simulink model "bramBurst_TransposeMatrix"  (R2021a)
settings: Solver=FixedStepDiscrete  StartTime=0.0  StopTime=44550*Ts  RelTol=1e-3
InitFcn:
  | matched_filter_fft_hdl_init;
model workspace (MAT data in the model file):
  mwTaskManagerKernelLatency = 0
  socvcb : containers.Map (value not decoded)
undefined symbols (not defined in the file or in its folder): columnWindowFun, DTsig_in, DTWindowFun, hdlbramBurst, N1, N2, radarDataCube, Ts
libraries: hdlsllib x35, simulink x11, dsphdlxfrm x1, dsphdlfiltering x1
(part 2 of 2)

== system bramBurst_TransposeMatrix/XDF/MatrixTranspose/addressControl/DDRbaseAddrCalc ==
  baseAddr : Inport
  ddrBank : Inport  Port=2
  Add : Sum  OutDataTypeStr=uint32
  Constant : Constant  Value=(N1 * N2 * hdlbramBurst.pAXIDataWidthBytes)  OutDataTypeStr=uint32  SampleTime=-1
  Switch1 : Switch  Criteria=u2 ~= 0
  Switch2 : Switch  Criteria=u2 ~= 0
  ddrWrAddr : Outport
  ddrRdAddr : Outport  Port=2
  wires:
  Constant/1 -> Add/1
  Add/1 -> Switch2/3, Switch1/1
  Switch1/1 -> ddrWrAddr/1
  ddrBank/1 -> Switch2/2, Switch1/2
  baseAddr/1 -> Switch2/1, Switch1/3, Add/2
  Switch2/1 -> ddrRdAddr/1

== system bramBurst_TransposeMatrix/XDF/MatrixTranspose/addressControl/ping_pong ==
  note: if 0 is selected then use first bank (starting at address 0) to read from
      | if 1 is selected then use the second bank (starting at offset) to read from
  ddrDone : Inport
  Logical Operator9 : Logic  Operator=XOR  IconShape=distinctive  AllPortsSameDT=off  OutDataTypeStr=boolean
  Unit Delay1 : UnitDelay  SampleTime=-1  HasFrameUpgradeWarning=on
  sr_latch : Subsystem
  ddrBank : Outport  VectorParamsAs1DForOutWhenUnconnected=off
  wires:
  Unit Delay1/1 -> Logical Operator9/1
  Logical Operator9/1 -> sr_latch/1(S)
  ddrDone/1 -> sr_latch/2(R), Logical Operator9/2
  sr_latch/1(Q) -> Unit Delay1/1, ddrBank/1  "DDR_BankSelect"

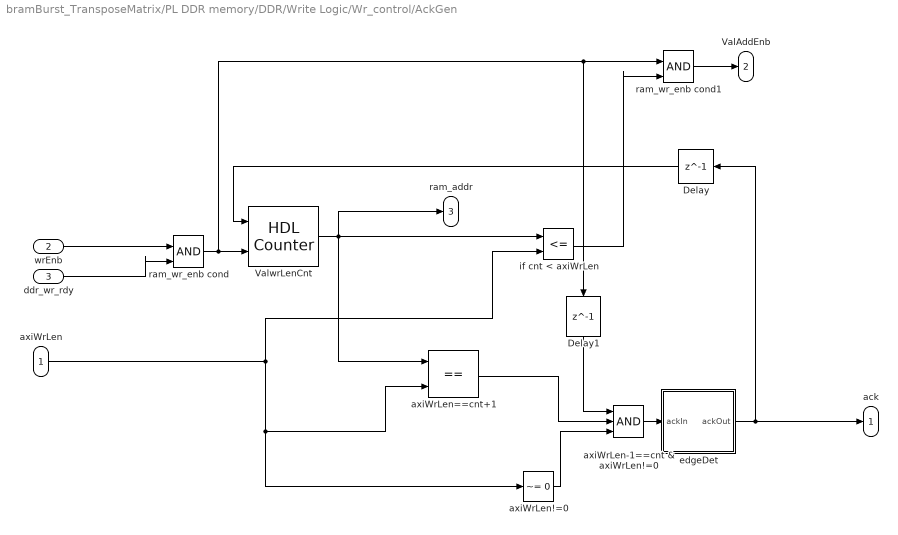
== system bramBurst_TransposeMatrix/PL DDR memory/DDR/Write Logic/Wr_control/AckGen ==
  axiWrLen : Inport
  wrEnb : Inport  Port=2
  ddr_wr_rdy : Inport  Port=3
  Delay : Delay  DelayLength=1
  Delay1 : Delay  DelayLength=1
  ValwrLenCnt : hdlsllib/Sources/HDL Counter  CountType=Free running  CountInit=0  CountStep=1  CountMax=25  CountFromType=Initial value  CountFrom=0  CountResetPort=on  CountLoadPort=off  CountEnbPort=on  CountDirPort=off  CountHitOutputPort=off  CountDataType=Unsigned  CountWordLen=32  CountFracLen=0  CountSampTime=1
  axiWrLen!=0 : simulink/Logic and Bit Operations/Compare To Constant  relop=~=  const=0  OutDataTypeStr=boolean
  "axiWrLen-1==cnt & axiWrLen!=0 " : Logic  Inputs=3  IconShape=distinctive  AllPortsSameDT=off  OutDataTypeStr=boolean
  axiWrLen==cnt+1 : RelationalOperator  Operator===  OutDataTypeStr=boolean  RndMeth=Nearest
  edgeDet : Subsystem
  if cnt < axiWrLen : RelationalOperator  Operator=<=  OutDataTypeStr=boolean  RndMeth=Nearest
  ram_wr_enb cond : Logic  IconShape=distinctive  AllPortsSameDT=off  OutDataTypeStr=boolean
  ram_wr_enb cond1 : Logic  IconShape=distinctive  AllPortsSameDT=off  OutDataTypeStr=boolean
  ack : Outport  VectorParamsAs1DForOutWhenUnconnected=off
  ValAddEnb : Outport  Port=2  VectorParamsAs1DForOutWhenUnconnected=off
  ram_addr : Outport  Port=3  VectorParamsAs1DForOutWhenUnconnected=off
  wires:
  Delay1/1 -> "axiWrLen-1==cnt & axiWrLen!=0 "/1
  Delay/1 -> ValwrLenCnt/1
  ram_wr_enb cond1/1 -> ValAddEnb/1
  ram_wr_enb cond/1 -> ValwrLenCnt/2, Delay1/1, ram_wr_enb cond1/1
  ddr_wr_rdy/1 -> ram_wr_enb cond/2
  ValwrLenCnt/1 -> ram_addr/1, if cnt < axiWrLen/1, axiWrLen==cnt+1/1
  axiWrLen/1 -> if cnt < axiWrLen/2, axiWrLen!=0/1, axiWrLen==cnt+1/2
  if cnt < axiWrLen/1 -> ram_wr_enb cond1/2
  wrEnb/1 -> ram_wr_enb cond/1
  axiWrLen!=0/1 -> "axiWrLen-1==cnt & axiWrLen!=0 "/3
  axiWrLen==cnt+1/1 -> "axiWrLen-1==cnt & axiWrLen!=0 "/2
  edgeDet/1(ackOut) -> Delay/1, ack/1
  "axiWrLen-1==cnt & axiWrLen!=0 "/1 -> edgeDet/1(ackIn)

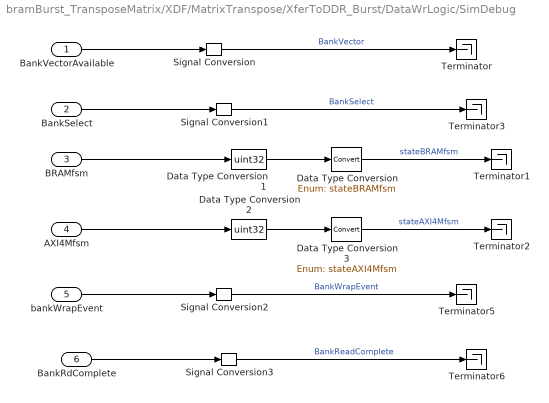
== system bramBurst_TransposeMatrix/XDF/MatrixTranspose/XferToDDR_Burst/DataWrLogic/SimDebug ==
  BankVectorAvailable : Inport
  BankSelect : Inport  Port=2
  BRAMfsm : Inport  Port=3
  AXI4Mfsm : Inport  Port=4
  bankWrapEvent : Inport  Port=5
  BankRdComplete : Inport  Port=6
  Data Type Conversion : DataTypeConversion  OutDataTypeStr=Enum: stateBRAMfsm
  Data Type Conversion1 : DataTypeConversion  OutDataTypeStr=uint32
  Data Type Conversion2 : DataTypeConversion  OutDataTypeStr=uint32
  Data Type Conversion3 : DataTypeConversion  OutDataTypeStr=Enum: stateAXI4Mfsm
  Signal Conversion{,1..3} (4 alike) : SignalConversion  OverrideOpt=off
  Terminator{,1..3,5..6} (6 alike) : Terminator
  wires:
  Signal Conversion/1 -> Terminator/1  "BankVector"
  Data Type Conversion2/1 -> Data Type Conversion3/1
  Data Type Conversion3/1 -> Terminator2/1  "stateAXI4Mfsm"
  Signal Conversion2/1 -> Terminator5/1  "BankWrapEvent"
  Data Type Conversion1/1 -> Data Type Conversion/1
  Signal Conversion3/1 -> Terminator6/1  "BankReadComplete"
  Signal Conversion1/1 -> Terminator3/1  "BankSelect"
  Data Type Conversion/1 -> Terminator1/1  "stateBRAMfsm"
  BRAMfsm/1 -> Data Type Conversion1/1
  AXI4Mfsm/1 -> Data Type Conversion2/1
  BankVectorAvailable/1 -> Signal Conversion/1
  bankWrapEvent/1 -> Signal Conversion2/1
  BankRdComplete/1 -> Signal Conversion3/1
  BankSelect/1 -> Signal Conversion1/1

== system bramBurst_TransposeMatrix/XDF/MatrixTranspose/XferToDDR_Burst/DataWrLogic/Subsystem ==
  wrctrlOut : Inport
  bankRdComplete : Inport  Port=2
  FIFO_backpressure_applied : Inport  Port=3
  <wr_complete> : Inport  Port=4
  In5 : Inport  Port=5
  Bit Concat : hdlsllib/Logic and Bit Operations/Bit Concat  numInputs=2
  Bus Selector1 : BusSelector  OutputSignals=wr_valid
  DebugBus : BusCreator  Inputs=5
  Demux : Demux  Outputs=2
  Detect Increase : simulink/Logic and Bit Operations/Detect Increase  vinit=0.0  OutDataTypeStr=boolean
  HDL Counter{,1..3} (4 alike) : hdlsllib/Sources/HDL Counter  CountType=Free running  CountInit=0  CountStep=1  CountMax=25  CountFromType=Initial value  CountFrom=0  CountResetPort=off  CountLoadPort=off  CountEnbPort=on  CountDirPort=off  CountHitOutputPort=off  CountDataType=Unsigned  CountWordLen=32  CountFracLen=0  CountSampTime=1
  Logical Operator1 : Logic  Operator=NOT  AllPortsSameDT=off  OutDataTypeStr=boolean
  debugRd : Outport
  wires:
  wrctrlOut/1 -> Bus Selector1/1
  FIFO_backpressure_applied/1 -> Logical Operator1/1
  HDL Counter2/1 -> DebugBus/1  "wr_complete_counter"
  <wr_complete>/1 -> HDL Counter2/1
  bankRdComplete/1 -> Detect Increase/1
  DebugBus/1 -> debugRd/1
  HDL Counter3/1 -> DebugBus/2  "bankCompleteCounter"
  Logical Operator1/1 -> HDL Counter/1
  HDL Counter/1 -> DebugBus/3  "FIFO_back_pressure_applied"
  Bus Selector1/1 -> HDL Counter1/1  "<wr_valid>"
  Detect Increase/1 -> HDL Counter3/1
  HDL Counter1/1 -> DebugBus/4  "CountWriteValids"
  In5/1 -> Demux/1
  Demux/1 -> Bit Concat/1
  Demux/2 -> Bit Concat/2
  Bit Concat/1 -> DebugBus/5  "FSM_read"

== system bramBurst_TransposeMatrix/XDF/MatrixTranspose/addressControl/ping_pong/sr_latch ==
  S : Inport
  R : Inport  Port=2
  Logical Operator1 : Logic  IconShape=distinctive  AllPortsSameDT=off  OutDataTypeStr=boolean
  Logical Operator2 : Logic  Operator=NOT  IconShape=distinctive  AllPortsSameDT=off  OutDataTypeStr=boolean
  Logical Operator9 : Logic  Operator=OR  IconShape=distinctive  AllPortsSameDT=off  OutDataTypeStr=boolean
  Unit Delay1 : UnitDelay  SampleTime=-1  HasFrameUpgradeWarning=on
  Q : Outport  VectorParamsAs1DForOutWhenUnconnected=off
  wires:
  Logical Operator9/1 -> Q/1, Unit Delay1/1
  Unit Delay1/1 -> Logical Operator1/2
  S/1 -> Logical Operator9/1
  R/1 -> Logical Operator2/1
  Logical Operator2/1 -> Logical Operator1/1
  Logical Operator1/1 -> Logical Operator9/2

== system bramBurst_TransposeMatrix/PL DDR memory/DDR/Write Logic/Wr_control/AckGen/edgeDet ==
  ackIn : Inport
  " ackIn==1" : simulink/Logic and Bit Operations/Compare To Constant  relop===  const=1  OutDataTypeStr=boolean
  ackIn Posedge Detect : Logic  IconShape=distinctive  AllPortsSameDT=off  OutDataTypeStr=boolean
  ackIn_d1 : Delay  DelayLength=1
  ackIn_d1==0 : simulink/Logic and Bit Operations/Compare To Constant  relop===  const=0  OutDataTypeStr=boolean
  ackOut : Outport  VectorParamsAs1DForOutWhenUnconnected=off
  wires:
  ackIn/1 -> ackIn_d1/1, " ackIn==1"/1
  ackIn_d1/1 -> ackIn_d1==0/1
  ackIn Posedge Detect/1 -> ackOut/1
  ackIn_d1==0/1 -> ackIn Posedge Detect/1
  " ackIn==1"/1 -> ackIn Posedge Detect/2

== matlab function bramBurst_TransposeMatrix/PL DDR memory/DDR/DDR Memory ==
  data: wr_din input INTERFACE_DT size=[INTERFACE_NUM_WORDS 1]; rd_dout output INTERFACE_DT size=[1 INTERFACE_NUM_WORDS]; wr_addr input; wr_en input; rd_addr input; INIT_DATA parameter; DDR_SIZE parameter; INIT_ADDR parameter; INTERFACE_WORD_LENGTH parameter; mem_data output; INTERFACE_NUM_WORDS parameter
function [rd_dout, mem_data] = ddr_memory(wr_din,wr_addr,wr_en,rd_addr,...
    INIT_DATA, DDR_SIZE, INIT_ADDR, INTERFACE_WORD_LENGTH, INTERFACE_NUM_WORDS)

DATA_NUM_BYTES = dataNumBytes(wr_din);

persistent mem
if isempty(mem)
    mem = zeros([1 DDR_SIZE],'uint8');
    if ~isempty(INIT_DATA)
        init_data_u8 = dataToBytes(INIT_DATA);
        idx = (1:numel(init_data_u8)) + INIT_ADDR;
        mem(idx) = init_data_u8;
    end
end

persistent rd_dout_reg
if isempty(rd_dout_reg)
    rd_dout_reg = zeros([1 INTERFACE_NUM_WORDS],'like',wr_din);
end

rd_dout = rd_dout_reg;

% READ update
rd_idx = (1:DATA_NUM_BYTES) + double(rd_addr);
if (rd_idx(end) > DDR_SIZE)
    error('Read from address 0x%X exceeds memory size.',uint32(rd_addr))
end
mem_rd_bytes = mem(rd_idx);
rd_dout_temp = zeros([1 INTERFACE_NUM_WORDS],'like',wr_din);
rd_dout_temp(:) = bytesToData(mem_rd_bytes, coder.const(INTERFACE_WORD_LENGTH));
% bytesToData
% if INTERFACE_WORD_LENGTH == 128
%     temp = typecast(mem_rd_bytes,'uint64');
%     temp1 = reshape(temp,2,[]);
%     rd_dout_temp(:)  = sim2fi(temp1, 0,128,0);
% else
%     rd_dout_temp(:)  = typecast(mem_rd_bytes,sprintf('uint%d',INTERFACE_WORD_LENGTH));
% end

rd_dout_reg = rd_dout_temp;

% WRITE update
if wr_en
    wr_idx = (1:DATA_NUM_BYTES) + double(wr_addr);
    if (wr_idx(end) > DDR_SIZE)
        error('Write from address 0x%X exceeds memory size.',uint32(wr_addr))
    end
    mem(wr_idx) = dataToBytes(wr_din);
end

mem_data = mem;

end

function dout = dataToBytes(din)
    temp1 = reshape(din,[],1); % force column vector
    if isfi(din)
        temp2 = reshape(fi2sim(temp1),[],1);
    else
        temp2 = temp1;
    end
    dout = typecast(temp2,'uint8');
end

function dout = bytesToData(din,wordLength)
    if wordLength == 128
        temp = typecast(din,'uint64');
        temp1 = reshape(temp,2,[]);
        dout = sim2fi(temp1, 0,128,0);
    else
        dout = typecast(din,sprintf('uint%d',wordLength));
    end
end

function val = dataNumBytes(din)
    temp = dataToBytes(din(1));
    val = numel(temp)*numel(din);
end

== matlab function bramBurst_TransposeMatrix/PL DDR memory/DDR/Read Logic/rd_control ==
  data: axi_rd_add input; axi_rd_len input; axi_rd_val input; axi_rd_ready input; ram_rd_addr output; ram_rd_val output boolean; toggle parameter; isDoneRead output; StateMachineOut output; ADDR_BIT_SHIFT parameter
function [ram_rd_addr, ram_rd_val,isDoneRead,StateMachineOut] = rd_add_gen(axi_rd_add,axi_rd_len, axi_rd_val,axi_rd_ready,toggle,ADDR_BIT_SHIFT)

%%%%%%%%%%%%%%%%%%%%%%%%%%%%%%%%%%%%%%%%%%%%%%%%%%%%%%
%%%Reg declaration
%RAM address generation counter
persistent ram_rd_cnt StateMachine
isDoneRead = false;
if(isempty(ram_rd_cnt))
    ram_rd_cnt = 0;
    StateMachine = uint32(0);
end


%read response ack
persistent reg_rd_ack;

if(isempty(reg_rd_ack))
    reg_rd_ack = false;
end

%read status
persistent rd_progress;

if(isempty(rd_progress))
    rd_progress = false;
end

%read addr valid flag 
persistent rd_addr_val;

if(isempty(rd_addr_val))
    rd_addr_val = false;
end

%read addr valid flag 
persistent rd_addr_val_toggle;

if(isempty(rd_addr_val_toggle))
    rd_addr_val_toggle = false;
end

%start address and length of read burst latch
persistent start_addr;
if(isempty(start_addr))
    start_addr = 0;
end

persistent leng_latch;
if(isempty(leng_latch))
    leng_latch = 1;
end

%%%%%%%%%%%%%%%%%%%%%%%%%%%%%%%%%%%%%%%%%%%%%%%
%output
ram_rd_addr = uint32(ram_rd_cnt);
ram_rd_val = rd_addr_val;
%%%%%%%%%%%%%%%%%%%%%%%%%%%%%%%%%%%%%%%%%%%%%%%
if((reg_rd_ack == true)&&(axi_rd_ready == true))
    ram_rd_cnt(:) = start_addr; %DAREN: This state looks like it is meant to init counter
    rd_addr_val = true;
    rd_addr_val_toggle = true; % TCM: Added to avoid valid low on 2nd cycle
    StateMachine(:) = 2;
elseif((rd_progress == true)&&(axi_rd_ready == true))
    StateMachine(:) = 3;
    if(rd_addr_val_toggle == true)
       ram_rd_cnt = ram_rd_cnt + 1;
       rd_addr_val = true;
    else
       rd_addr_val = false;
   
    end
    if(toggle)
       rd_addr_val_toggle = ~(rd_addr_val_toggle);
    else
       rd_addr_val_toggle = true;
    end
    if ram_rd_cnt == leng_latch-2
            isDoneRead = true;
    end
    
elseif((rd_progress == false))  
    StateMachine(:) = 11; % DAREN: Post read progress
    ram_rd_cnt = 0;
    rd_addr_val = false;
else
    StateMachine(:) = 12; % DAREN: for handling back-pressure
    rd_addr_val = false;
end


%read progress flag
if((reg_rd_ack)&&((ram_rd_cnt-start_addr)<(leng_latch-1)))
    rd_progress = true;
%     StateMachine = 2;
   
elseif((ram_rd_cnt-start_addr)==(leng_latch-1))
    StateMachine(:) = 10; % DAREN: Counter has completed read
    rd_progress = false;
    isDoneRead = true; 
end


%start address , length of burst latching
if(axi_rd_val)
    leng_latch(:) = axi_rd_len;
    start_addr(:) = bitshift(axi_rd_add,-ADDR_BIT_SHIFT);
    reg_rd_ack = true;
    StateMachine(:) = 1;
elseif rd_progress == false
    isDoneRead = true;
    reg_rd_ack = false;
else
    reg_rd_ack = false;
 
end
StateMachineOut = uint32(0);
StateMachineOut(:) = StateMachine;

== matlab function bramBurst_TransposeMatrix/PL DDR memory/DDR/Write Logic/Wr_control/MATLAB Function ==
  data: axi_wr_en input; wr_leng output; axi_wr_length input; wr_ack input
function wr_leng = addr_latch(axi_wr_en,axi_wr_length,wr_ack)
%#codegen

persistent axi_wr_en_d1;
if(isempty(axi_wr_en_d1))
axi_wr_en_d1 = false;
end

persistent reg_len;
if(isempty(reg_len))
    reg_len = fi(0,0,32,0);%uint32(0);
end


persistent reg_len_d1;
if(isempty(reg_len_d1))
    reg_len_d1 = fi(0,0,32,0);%uint32(0);
end

reg_len_d1 = reg_len;
wr_leng = reg_len;

if((axi_wr_en==true)&&(axi_wr_en_d1==false)&&(reg_len_d1==0)) 
  reg_len= fi(axi_wr_length,0,32,0);%axi_wr_length;
elseif(wr_ack)
  reg_len= fi(0,0,32,0);%uint32(0);    
end

axi_wr_en_d1 = axi_wr_en;

== matlab function bramBurst_TransposeMatrix/PL DDR memory/DDR/Write DDR Data to Workspace/Save to Workspace ==
  data: data input; save parameter; varname parameter
function save_to_workspace(data,save,varname)

coder.extrinsic('assignin')

if save
    assignin('base',char(varname),data);
end

== matlab function bramBurst_TransposeMatrix/XDF/MatrixTranspose/XferToDDR_Burst/DataWrLogic/MLFB ==
  data: bramWrData output; bramWrAddr output; bramWrEnb output; bramRdAddr output; WrCtrlO output Bus: BusAXIWriteCtrlM2S; ddr_write_done output; axis_ready_o output; dataIn input; validIn input; WrCtrlI input; baseAddr input; debug_BankRdVector output; debug_BankSelect output; debug_BRAMFsm output; pNumCols parameter; pNumRows parameter; pMaxBankLines parameter; pMaxNumBanks parameter; pAXIDataWidthBytes parameter; debug_AXI4MFsm output; debug_wrapBRAMBank output; debug_BankReadComplete output; pBramAddrWidth parameter; debug_readyOverride output
function [bramWrData, bramWrAddr, bramWrEnb, bramRdAddr, WrCtrlO, ddr_write_done, axis_ready_o, debug_BankRdVector,...
          debug_BankSelect, debug_BRAMFsm, debug_AXI4MFsm, debug_wrapBRAMBank, debug_BankReadComplete, debug_readyOverride] =  ...
burstTranspose(dataIn, validIn, WrCtrlI, baseAddr, pNumCols, pNumRows, pMaxBankLines, pMaxNumBanks, pAXIDataWidthBytes, pBramAddrWidth)

% define FSM States
IDLE = fi(0,0,4,0);
% States for managing the writing to BRAM
LINEBUFFER = fi(1,0,4,0);
LINESTART = fi(3,0,4,0);
% States for managing the writing to DDR
BURSTSTART = fi(1,0,4,0);
BURSTNEXT  = fi(3,0,4,0);
WAITBURSTCOMPLETE = fi(4,0,4,0);
WAITBURSTREADY = fi(5,0,4,0);
WAITONBANKRDY =fi(2,0,4,0);

persistent stateBRAMfsm burstState WrBank RdBank WrData BankRdy...
           WrAddr RdAddr WrEnb colCnt rowCnt WrBankLine RdBankLine...
           WrDone aximWrAddr aximWrValid startRdAddr burstCount...
           aximWrLen aximNumRowsWritten bankWrWrap...
           aximm2s_ready ready_override
           
 
if isempty(stateBRAMfsm)
    stateBRAMfsm = IDLE;
    burstState = IDLE;
    bankWrWrap = false;
    WrBank = fi(0,0,8,0);
    RdBank = fi(0,0,8,0);
    BankRdy = zeros(uint32(pMaxNumBanks),1,'logical');
    WrBankLine = uint16(0);
    RdBankLine = uint16(0);
    WrEnb = false;
    WrDone = false;
    aximWrAddr = uint32(0);
    aximWrLen = uint32(pMaxBankLines);
    aximWrValid = false;
    WrData = cast(0,'like', dataIn);
%     WrAddr = fi(0,0,14,0);
%     RdAddr = fi(0,0,14,0);
    WrAddr = fi(0,0,pBramAddrWidth,0);
    RdAddr = cast(0,'like',WrAddr);
    startRdAddr = cast(0,'like',WrAddr);
    burstCount = uint16(0);
    colCnt = fi(0,0,ceil(log2(pNumCols)),0);
    rowCnt = fi(0,0,ceil(log2(pNumRows)),0);
    aximNumRowsWritten = uint32(0);
    
    % additional ready signals
    aximm2s_ready = true;
    ready_override = true;
end


%% Assign outputs
bramWrData = WrData;
bramWrEnb = WrEnb;
bramWrAddr = WrAddr;
bramRdAddr = RdAddr;
wr_ddr_addr = uint32((aximWrAddr * pAXIDataWidthBytes) + baseAddr);
WrCtrlO = struct('wr_addr', wr_ddr_addr, 'wr_len', aximWrLen, 'wr_valid', aximWrValid);
ddr_write_done = WrDone;
WrDone = false;  % Note: WrDone true for one clock only


%% Ready conditions for axi4-stream
% if there is not enough banks available, check to see if all three are
if ~aximm2s_ready  && (bitconcat(fi(BankRdy,0,1,0)) == 0)
    aximm2s_ready = true;
end

% if ready_override == false
% aximm2s_ready = aximm2s_ready & ready_override;
% end

% if <condition that we are still reading> && (bitconcat(fi(BankRdy,0,1,0)) == 0)
%     aximm2s_ready = true;
% end


%% For debug outputs only
debug_BankRdVector = BankRdy; % display status of each BRAM bank. if a 1 is written to a bank, it means it  has data that has NOT been fully read out yet
debug_BankSelect = WrBank;  % which BRAM bank is selected to write new data to. Zero indexed
debug_wrapBRAMBank = bankWrWrap; % Will occur when we wrap to the first BRAM Bank
debug_BankReadComplete = (RdBankLine == 0); % finished reading a bank (got to end of column) and reset to zero event

debug_BRAMFsm = stateBRAMfsm; % BRAM write state machine
debug_AXI4MFsm = burstState;  % BRAM Read -> DDR4 state machine




%%

% process col and row counts
if WrEnb  % write to BRAM
%     fprintf("+BRAM: %08x @ %u Col %u Row %u WrBankLine %u WrBank %u\n", uint32(WrData), uint32(WrAddr), uint16(colCnt), uint16(rowCnt), WrBankLine, uint16(WrBank));
    if colCnt == pNumCols-1
        if rowCnt == pNumRows-1 % end of matrix
            BankRdy(WrBank+1) = true;
            WrBank(:) = WrBank + 1;
            if WrBank == pMaxNumBanks
                WrBank(:) = 0;
                WrAddr(:) = 0;
            end
            stateBRAMfsm = IDLE;
           
        else
            colCnt(:) = 0;
            rowCnt(:) = rowCnt + 1;
            WrBankLine(:) = WrBankLine + 1;
            if WrBankLine == pMaxBankLines
                BankRdy(WrBank+1) = true;
                if burstState == IDLE
                    burstState = BURSTSTART;
                    startRdAddr(:) = 0;
                end
                WrBankLine(:) = 0;
                WrBank(:) = WrBank + 1;
                % NOTE wrap around to bank 0 
                % The Number of banks might need to change to keep up with
                % the write to DDR rate - keep track of possible collision
                if WrBank == pMaxNumBanks
                    bankWrWrap = true;
                    WrBank(:) = 0;
                    WrAddr(:) = 0;
                end
                if  BankRdy(WrBank+1) == true
                   aximm2s_ready = false;
%                 else
%                    aximm2s_ready = true; 
%                     error('Bank Overrun! Increase number of available banks in BRAM.');
                end
            end
        end
    else
        colCnt(:) = colCnt + 1;
        
        if (colCnt == pNumCols-1) && (rowCnt == pNumRows-1)
             ready_override = false; % dont accept any more data until we are done
        end
    end
end

% reset these after every write
WrEnb = false;

% FSM to manage writing input data to BRAM
switch stateBRAMfsm
    case IDLE
        % first validIn could be on a later clock or on this clock
        if validIn
            WrAddr(:) = 0;
            colCnt(:) = 0;
            rowCnt(:) = 0;
            WrBank(:) = 0;
            BankRdy = zeros(uint32(pMaxNumBanks),1,'logical');
            WrBankLine(:) = 0;
            RdBank(:) = 0;
            
            WrData = dataIn;
            WrEnb = true;
            stateBRAMfsm = LINEBUFFER;
        end
    case LINESTART
        if validIn
            WrData = dataIn;
            WrEnb = true; 
            stateBRAMfsm = LINEBUFFER;
        end
    case LINEBUFFER
        if validIn
            if bankWrWrap
                WrAddr(:) = 0;
                bankWrWrap = false;
            else
                WrAddr(:) = WrAddr + 1;
            end
            WrData = dataIn;
            WrEnb = true; 
        end
end

% FSM To manage the Write to DDR in Bursts in maxBufLines
switch burstState
    case IDLE
    case BURSTSTART
        aximWrAddr(:) = 0; % (bank-1) * maxBufLines;
        RdAddr = startRdAddr ;
        burstCount(:) = 0;
        if BankRdy(RdBank+1) == true
            burstState = WAITBURSTREADY;
        else
            burstState = WAITONBANKRDY;
        end
    case WAITBURSTREADY
        if WrCtrlI.wr_ready
            aximWrValid = true;
            RdAddr(:) = RdAddr + pNumCols;
            burstState(:) = BURSTNEXT;
            burstCount(:) = burstCount + 1;
            if burstCount == aximWrLen
                burstState = WAITBURSTCOMPLETE;
                burstCount(:) = 0;
            end
        else
           aximWrValid = false;
        end
    case BURSTNEXT
        if WrCtrlI.wr_ready
            aximWrValid = true;
            RdAddr(:) = RdAddr + pNumCols;
            burstCount(:) = burstCount + 1;
            if burstCount == aximWrLen
                burstState = WAITBURSTCOMPLETE;
                burstCount(:) = 0;
            end
        else
            aximWrValid = false;
            burstState = WAITBURSTREADY;
        end
    case WAITBURSTCOMPLETE
        aximWrValid = false;
        if WrCtrlI.wr_complete
%         if WrCtrlI.wr_ready  % support pipelined writes (R2020a+)
            aximWrAddr(:) = aximWrAddr + pNumRows;
            % go to next burst of maxBufLines
            startRdAddr(:) = startRdAddr + 1; 
            burstState = WAITBURSTREADY;
            RdBankLine(:) = RdBankLine + 1;
            if RdBankLine == pNumCols   % Reached the end of a bank, need to move to next bank
                RdBankLine(:) = 0;
                BankRdy(RdBank+1) = false;
                RdBank(:) = RdBank + 1;
                if RdBank == pMaxNumBanks
                    RdBank(:) = 0;
                    startRdAddr(:) = 0;
                end
                startRdAddr(:) = uint16(RdBank) * coder.const((pNumCols * pMaxBankLines));  
                aximNumRowsWritten(:) = aximNumRowsWritten + aximWrLen;
                if (pNumRows - aximNumRowsWritten) < pMaxBankLines
                    aximWrLen(:) = pNumRows - aximNumRowsWritten;
                end
                aximWrAddr(:) = aximNumRowsWritten;
                if BankRdy(RdBank+1) == false
                    burstState = WAITONBANKRDY;
%                     fprintf('WAITING for Ready Bank: %u\n', uint32(RdBank));
                end
                if aximNumRowsWritten == pNumRows
                    aximWrLen = uint32(pMaxBankLines);
                    aximNumRowsWritten(:)  = 0;
                    burstState(:) = IDLE;
                    WrDone = true;
                    ready_override = true; % accept new data into BRAM now
                end
            end
            RdAddr(:) = startRdAddr; 
        end        
    case WAITONBANKRDY
        if BankRdy(RdBank+1) == true
            burstState = WAITBURSTREADY;
        end
end


axis_ready_o = aximm2s_ready ;
debug_readyOverride = ready_override;

== matlab function bramBurst_TransposeMatrix/ReadMatrixData ==
  data: signal_o output; valid_o output; MatrixInput parameter; ValidGap parameter; ready input; GapsInMatrix parameter
function [signal_o, valid_o] = fcn(MatrixInput,ValidGap, ready, GapsInMatrix)
persistent matrixReadState colCounter rowCounter gapCounter matrixReadCount

WAIT_FOR_READY = uint32(0);
READ_COLUMN = uint32(1);
ADD_GAP_AFTER_COLUMN = uint32(2);
SHUT_DOWN_STATE = uint32(3);

GAP_MAX = GapsInMatrix + ValidGap;

if isempty(matrixReadState)
    colCounter = uint32(1); % use 1 indexing
    rowCounter = uint32(1); 
    matrixReadState = WAIT_FOR_READY; 
    gapCounter = 0;
    matrixReadCount = uint32(0);
end

signal_o = cast(complex(0),'like',MatrixInput);
valid_o = false;
[numRow, numCol]= size(MatrixInput);
    
%% Read value from matrix
switch(matrixReadState)
    case(WAIT_FOR_READY)
        if ready
            matrixReadState(:) = READ_COLUMN;
        end            
        valid_o = false;
    case(READ_COLUMN) % this is reading along the column, row by row
        if ready
            signal_o = MatrixInput(rowCounter,colCounter);
            valid_o = true;
            
            if rowCounter < numRow
                rowCounter = rowCounter + 1;               
            else
                matrixReadState(:) = ADD_GAP_AFTER_COLUMN;                      
            end
        else
            matrixReadState(:) = WAIT_FOR_READY;
        end
    case(ADD_GAP_AFTER_COLUMN)
        if gapCounter < GAP_MAX
            gapCounter(:) = gapCounter(:) + 1;
        else
            gapCounter(:) = 0;
            matrixReadState(:) = READ_COLUMN;             
            if colCounter < numCol % 
                rowCounter(:) = 1;  % more columns left to cover, move to next one
                colCounter(:) = colCounter + 1;
                
%                 if matrixReadCount >= 1 && colCounter == 2 % if we are in the 2nd matrix and we just finished a column
%                     matrixReadState(:) = SHUT_DOWN_STATE;
%                 end
            else
%                 matrixReadState(:) = SHUT_DOWN_STATE;
                %end of matrix...
                rowCounter(:) = 1; 
                colCounter(:) = 1;  % Go back to beginning...
                matrixReadCount(:) = matrixReadCount(:) + 1;
            end                
        end
        valid_o = false;
    case(SHUT_DOWN_STATE)
        % dont do anything here 
        valid_o = false;
end

    
  
   
end

== matlab function bramBurst_TransposeMatrix/PL DDR memory/DDR/ddr_ready/READY generation ==
  data: ready output; BANDWIDTH_DERATING parameter
function ready = ready_gen(BANDWIDTH_DERATING)

FRAME_SIZE = coder.const(1000);

persistent rand_frame idx
if isempty(rand_frame)
    rand_frame = rand([FRAME_SIZE 1]);
    idx = 1;
end

ready = rand_frame(idx) > BANDWIDTH_DERATING;

if idx==FRAME_SIZE
    idx = 1;
    rand_frame = rand([FRAME_SIZE 1]);
else
    idx=idx+1;
end

== matlab function bramBurst_TransposeMatrix/PL DDR memory/DDR/Read Logic/axim_rd_aready_behavior ==
  data: rdDonePulse input; rd_rdy output; READ_DOWNTIME parameter
function rd_rdy = aready(rdDonePulse, READ_DOWNTIME)

persistent rdy_state delay_count
if isempty(rdy_state)
    rdy_state = uint32(0);
    delay_count = uint8(0);
end

STATE_IDLE = uint32(0);
STATE_WAIT = uint32(1);
rd_rdy = false;

switch(rdy_state)
    case(STATE_IDLE)
        if rdDonePulse % if a read just completed, wait a few moments
            rdy_state(:) = STATE_WAIT;            
        else
            rd_rdy = true;
        end
        
    case(STATE_WAIT)
        rd_rdy = false;
        
        if delay_count == READ_DOWNTIME
            delay_count(:) = 0;
            rdy_state(:) = STATE_IDLE;
        else
            delay_count(:) = delay_count + 1;
        end
    otherwise
        rd_rdy = false;        
end


end
